simulink model "SYS5_2"  (R2021b)
settings: Solver=VariableStepAuto  StartTime=0.0  StopTime=0.1  RelTol=1e-3  EnableMultiTasking=on
values from neighbouring files (symbols this model uses):
  Jn = 2*Jd    (= 0.000334)    [main.m]
  K = place(A,B,p)    [main.m]
  ke = (Un-R*In)/wn    (= 0.320333333333)    [main.m]
  km = Mn/In    (= 0.228971962617)    [main.m]
  ku = 20    [main.m]
  La = 10^-3 * 58    (= 0.058)    [main.m]
  R = 8.5    [main.m]
settings Model: Creator=Алекс  LastModifiedBy=vkad
settings SolverCC: AlgebraicLoopSolver=TrustRegion
settings DataIOCC: LimitDataPoints=on  SaveFormat=Array  SignalLoggingSaveFormat=ModelDataLogs  ReturnWorkspaceOutputs=off
settings OptimizationCC: ExpressionDepthLimit=2147483647  LifeSpan=inf
settings DebuggingCC: UnderspecifiedInitializationDetection=Classic  MergeDetectMultiDrivingBlocksExec=none  FcnCallInpInsideContextMsg=warning  StateNameClashWarn=warning  SFUnexpectedBacktrackingDiag=warning  SFNoUnconditionalDefaultTransitionDiag=warning  SFExecutionAtInitializationDiag=none  SFMachineParentedDataDiag=warning  ArithmeticOperatorsInVariantConditions=warning
settings HardwareCC: ProdBitPerPointer=32  ProdBitPerSizeT=32  ProdBitPerPtrDiffT=32  ProdLargestAtomicFloat=None  ProdIntDivRoundTo=Undefined  ProdEndianess=Unspecified  ProdWordSize=32  ProdHWDeviceType=32-bit Generic
settings ModelReferenceCC: PropagateSignalLabelsOutOfModel=off
settings SFSimCC: SimUseLocalCustomCode=off  CustomCodeUndefinedFunction=UseInterfaceOnly
settings RTWCC: RTWUseLocalCustomCode=off
settings CodeAppCC: StateflowObjectComments=on
settings GRTTargetCC: TargetLangStandard=C89/C90 (ANSI)  CombineOutputUpdateFcns=off  GRTInterface=on
settings ConfigComp: CovMetricSettings=dw  CovSaveCumulativeToWorkspaceVar=on  CovSaveSingleToWorkspaceVar=on  CovExternalEMLEnable=off  CovSFcnEnable=off

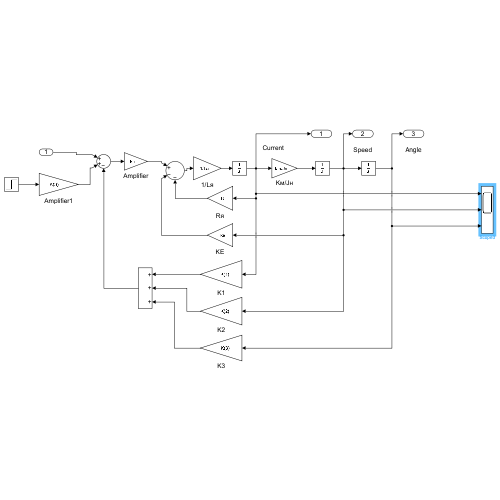
[thumbnail: Simulink's stored preview of the top-level diagram]
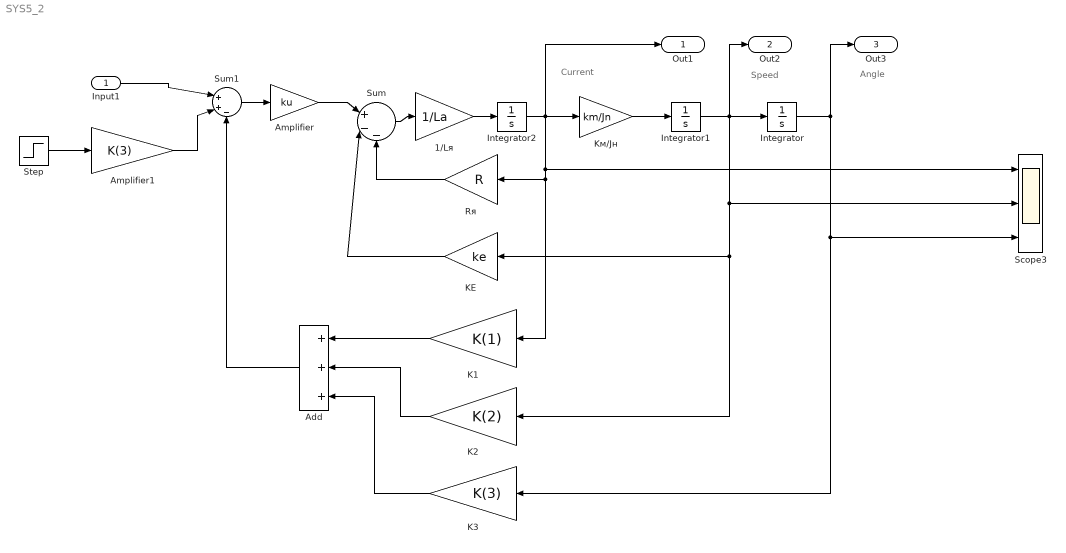
== system SYS5_2 ==
  note: Angle
  note: Speed
  note: Current
  Input1 : Inport
  1/Lя : Gain  Gain=1/La
  Add : Sum  Inputs=+++
  Amplifier : Gain  Gain=ku
  Amplifier1 : Gain  Gain=K(3)
  Integrator : Integrator
  Integrator1 : Integrator
  Integrator2 : Integrator
  K1 : Gain  Gain=K(1)
  K2 : Gain  Gain=K(2)
  K3 : Gain  Gain=K(3)
  KE : Gain  Gain=ke
  Kм/Jн : Gain  Gain=km/Jn
  Rя : Gain  Gain=R
  Scope3 : Scope  NumInputPorts=3
  Step : Step  Time=0  SampleTime=0
  Sum : Sum  Inputs=|+--
  Sum1 : Sum  Inputs=|++-
  Out1 : Outport  BusOutputAsStruct=on
  Out2 : Outport  Port=2  BusOutputAsStruct=on
  Out3 : Outport  Port=3  BusOutputAsStruct=on
  wires:
  Sum/1 -> 1/Lя/1
  Integrator1/1 -> Out2/1, Integrator/1, K2/1, KE/1, Scope3/2
  Integrator/1 -> Scope3/3, K3/1, Out3/1
  Kм/Jн/1 -> Integrator1/1
  Integrator2/1 -> Out1/1, Kм/Jн/1, Scope3/1, Rя/1, K1/1
  1/Lя/1 -> Integrator2/1
  Rя/1 -> Sum/3
  KE/1 -> Sum/2
  Input1/1 -> Sum1/1
  Sum1/1 -> Amplifier/1
  Amplifier/1 -> Sum/1
  Add/1 -> Sum1/3
  Amplifier1/1 -> Sum1/2
  Step/1 -> Amplifier1/1
  K1/1 -> Add/1
  K2/1 -> Add/2
  K3/1 -> Add/3
